simulink model "nwlr3"  (R2024a)
settings: Solver=VariableStepAuto  StartTime=0.0  StopTime=500  RelTol=1e-3
settings Model: Creator=Макс  LastModifiedBy=Григорий

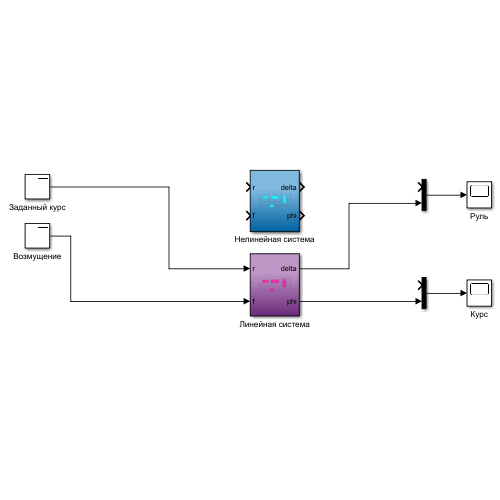
[thumbnail: Simulink's stored preview of the top-level diagram]
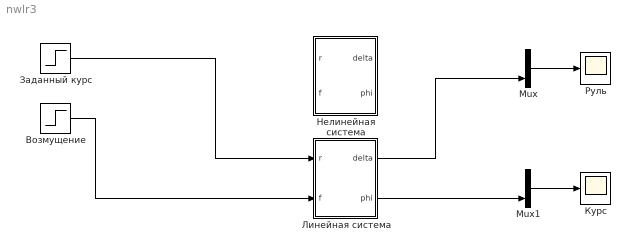
== system nwlr3 ==
  Mux : Mux  Inputs=2
  Mux1 : Mux  Inputs=2
  Возмущение : Step  Time=0  After=0  SampleTime=0
  Заданный курс : Step  Time=0  After=10  SampleTime=0
  Курс : Scope
  Линейная система : Subsystem
  Нелинейная система : Subsystem
  Руль : Scope
  wires:
  Заданный курс/1 -> Линейная система/1(r)
  Возмущение/1 -> Линейная система/2(f)
  Mux1/1 -> Курс/1
  Mux/1 -> Руль/1
  Линейная система/1(delta) -> Mux/2
  Линейная система/2(phi) -> Mux1/2

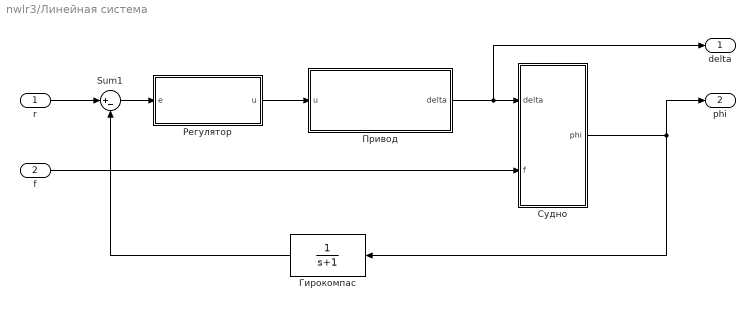
== system nwlr3/Линейная система ==
  r : Inport
  f : Inport  Port=2
  Sum1 : Sum  Inputs=|+-
  Гирокомпас : TransferFcn  Denominator=[1 1]
  Привод : Subsystem
  Регулятор : Subsystem
  Судно : Subsystem
  delta : Outport
  phi : Outport  Port=2
  wires:
  f/1 -> Судно/2(f)
  Sum1/1 -> Регулятор/1(e)
  r/1 -> Sum1/1
  Судно/1(phi) -> phi/1, Гирокомпас/1
  Привод/1(delta) -> delta/1, Судно/1(delta)
  Гирокомпас/1 -> Sum1/2
  Регулятор/1(u) -> Привод/1(u)

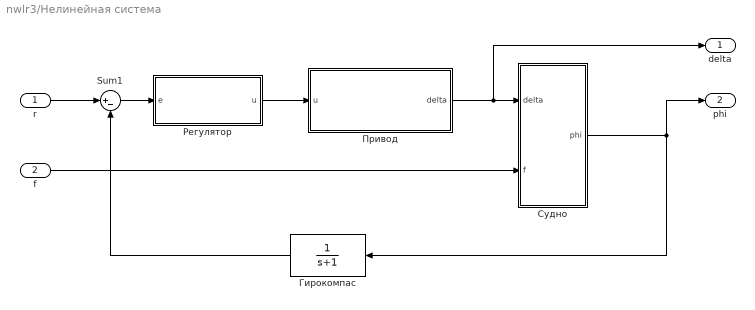
== system nwlr3/Нелинейная система ==
  r : Inport
  f : Inport  Port=2
  Sum1 : Sum  Inputs=|+-
  Гирокомпас : TransferFcn  Denominator=[1 1]
  Привод : Subsystem
  Регулятор : Subsystem
  Судно : Subsystem
  delta : Outport
  phi : Outport  Port=2
  wires:
  Судно/1(phi) -> phi/1, Гирокомпас/1
  Гирокомпас/1 -> Sum1/2
  Регулятор/1(u) -> Привод/1(u)
  Привод/1(delta) -> delta/1, Судно/1(delta)
  Sum1/1 -> Регулятор/1(e)
  r/1 -> Sum1/1
  f/1 -> Судно/2(f)

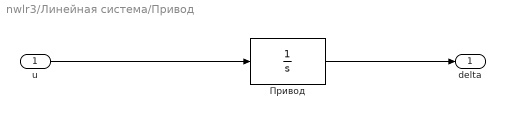
== system nwlr3/Линейная система/Привод ==
  u : Inport
  Привод : TransferFcn  Tag=Привод  Denominator=[1 0]
  delta : Outport
  wires:
  Привод/1 -> delta/1
  u/1 -> Привод/1

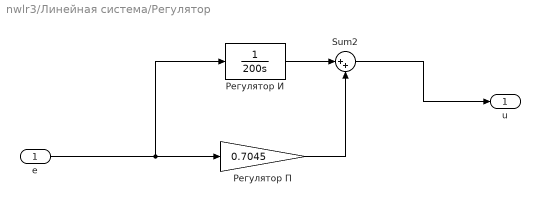
== system nwlr3/Линейная система/Регулятор ==
  e : Inport
  Sum2 : Sum  Inputs=|++
  Регулятор И : TransferFcn  Denominator=[200 0]
  Регулятор П : Gain  Gain=0.7045
  u : Outport
  wires:
  Регулятор П/1 -> Sum2/2
  Регулятор И/1 -> Sum2/1
  e/1 -> Регулятор И/1, Регулятор П/1
  Sum2/1 -> u/1

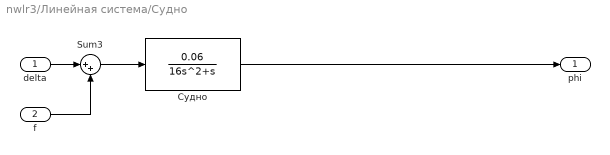
== system nwlr3/Линейная система/Судно ==
  delta : Inport
  f : Inport  Port=2
  Sum3 : Sum  Inputs=|++
  Судно : TransferFcn  Numerator=[0.06]  Denominator=[16 1 0]
  phi : Outport
  wires:
  f/1 -> Sum3/2
  Sum3/1 -> Судно/1
  delta/1 -> Sum3/1
  Судно/1 -> phi/1

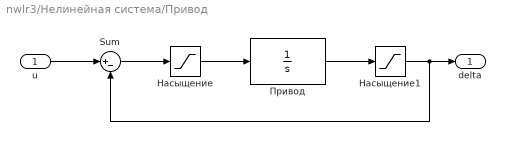
== system nwlr3/Нелинейная система/Привод ==
  u : Inport
  Sum : Sum  Inputs=|+-
  Насыщение : Saturate  UpperLimit=3  LowerLimit=-3
  Насыщение1 : Saturate  UpperLimit=30  LowerLimit=-30
  Привод : TransferFcn  Tag=Привод  Denominator=[1 0]
  delta : Outport
  wires:
  Насыщение1/1 -> Sum/2, delta/1
  Привод/1 -> Насыщение1/1
  Насыщение/1 -> Привод/1
  Sum/1 -> Насыщение/1
  u/1 -> Sum/1

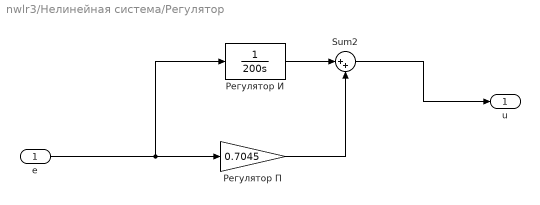
== system nwlr3/Нелинейная система/Регулятор ==
  e : Inport
  Sum2 : Sum  Inputs=|++
  Регулятор И : TransferFcn  Denominator=[200 0]
  Регулятор П : Gain  Gain=0.7045
  u : Outport
  wires:
  Регулятор П/1 -> Sum2/2
  Регулятор И/1 -> Sum2/1
  e/1 -> Регулятор И/1, Регулятор П/1
  Sum2/1 -> u/1

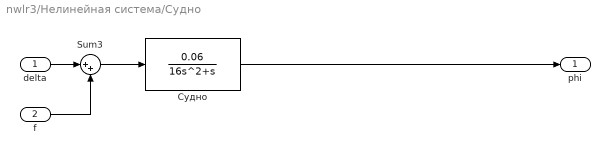
== system nwlr3/Нелинейная система/Судно ==
  delta : Inport
  f : Inport  Port=2
  Sum3 : Sum  Inputs=|++
  Судно : TransferFcn  Numerator=[0.06]  Denominator=[16 1 0]
  phi : Outport
  wires:
  f/1 -> Sum3/2
  Sum3/1 -> Судно/1
  delta/1 -> Sum3/1
  Судно/1 -> phi/1
